simulink model "Pendulum_final"  (R2024b)
settings: Solver=VariableStepAuto  StartTime=0.0  StopTime=10.0  RelTol=1e-3
values from neighbouring files (symbols this model uses):
  K = lqr(A_upper,B_upper,Q,R)    [main_final.m]
  P1 = - 0.7065    (= -0.7065)    [main_final.m]
  P2 = - 1.44    (= -1.44)    [main_final.m]
  P3 = 0.05622    [main_final.m]
  P4 = 0.008979    [main_final.m]
  P5 = 0.00232    [main_final.m]
  P6 = 1    [main_final.m]
  phi_dot_dot_sat = 100    [main_final.m]
  phi_dot_dot_threshold = 1e-10    [main_final.m]
  tau_a_sat = inf    [main_final.m]
  tau_a_threshold = 1e-10    [main_final.m]
  theta_dot_dot_sat = 100    [main_final.m]
  theta_dot_dot_threshold = 1e-10    [main_final.m]
settings Model: Creator=louis  LastModifiedBy=sipak

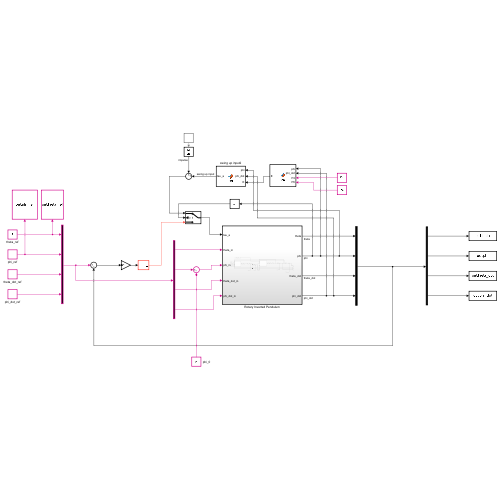
[thumbnail: Simulink's stored preview of the top-level diagram]
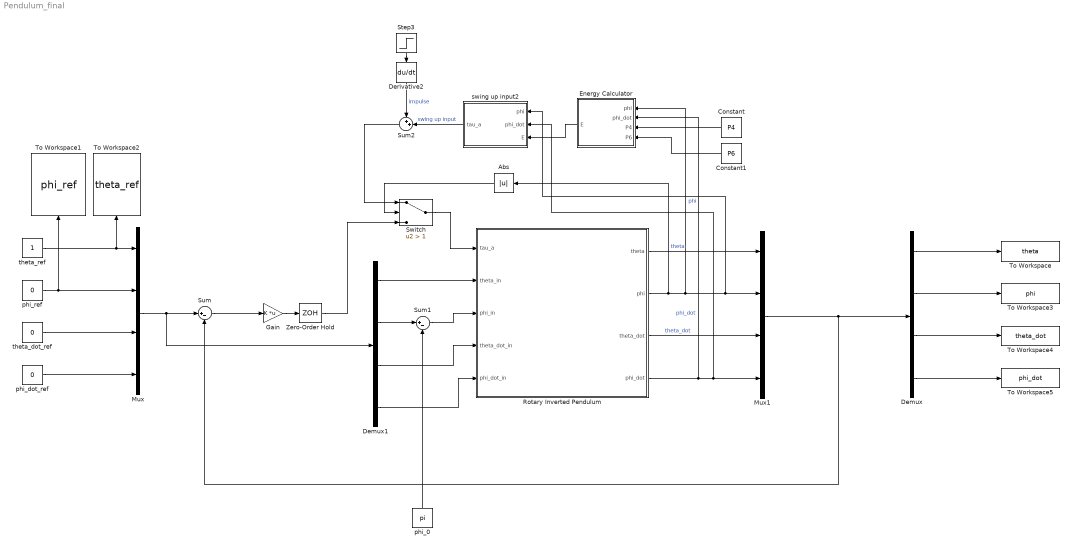
== system Pendulum_final ==
  Abs : Abs  SaturateOnIntegerOverflow=off
  Constant : Constant  Value=P4
  Constant1 : Constant  Value=P6
  Demux : Demux
  Demux1 : Demux
  Derivative2 : Derivative
  Energy Calculator : MATLAB Function  TreatAsAtomicUnit=on
  Gain : Gain  Gain=K  Multiplication=Matrix(K*u)
  Mux : Mux
  Mux1 : Mux
  Rotary Inverted Pendulum : Subsystem
  Step3 : Step  SampleTime=0
  Sum : Sum  Inputs=|+-
  Sum1 : Sum  Inputs=|+-
  Sum2 : Sum  Inputs=++|
  Switch : Switch  Criteria=u2 > Threshold  Threshold=1  SaturateOnIntegerOverflow=off  InputSameDT=off
  To Workspace : ToWorkspace  VariableName=theta  SampleTime=-1
      settings: Save2DSignal=2-D array (concatenate along first dimension)
  To Workspace1 : ToWorkspace  VariableName=phi_ref  SampleTime=-1
      settings: Save2DSignal=2-D array (concatenate along first dimension)
  To Workspace2 : ToWorkspace  VariableName=theta_ref  SampleTime=-1
  To Workspace3 : ToWorkspace  VariableName=phi  SampleTime=-1
  To Workspace4 : ToWorkspace  VariableName=theta_dot  SampleTime=-1
  To Workspace5 : ToWorkspace  VariableName=phi_dot  SampleTime=-1
  Zero-Order Hold : ZeroOrderHold  SampleTime=0.01
  phi_0 : Constant  Value=pi
  phi_dot_ref : Constant  Value=0
  phi_ref : Constant  Value=0
  swing up input2 : MATLAB Function  TreatAsAtomicUnit=on
  theta_dot_ref : Constant  Value=0
  theta_ref : Constant
  wires:
  theta_dot_ref/1 -> Mux/3
  phi_ref/1 -> Mux/2, To Workspace1/1
  theta_ref/1 -> Mux/1, To Workspace2/1
  Gain/1 -> Zero-Order Hold/1
  Mux/1 -> Demux1/1, Sum/1
  Mux1/1 -> Demux/1, Sum/2
  Sum/1 -> Gain/1
  Demux/1 -> To Workspace/1
  Demux/2 -> To Workspace3/1
  Demux/3 -> To Workspace4/1
  Demux/4 -> To Workspace5/1
  Demux1/3 -> Rotary Inverted Pendulum/4(theta_dot_in)
  Demux1/4 -> Rotary Inverted Pendulum/5(phi_dot_in)
  Demux1/1 -> Rotary Inverted Pendulum/2(theta_in)
  Rotary Inverted Pendulum/1(theta) -> Mux1/1  "theta"
  Rotary Inverted Pendulum/2(phi) -> Abs/1, swing up input2/1(phi), Mux1/2, Energy Calculator/1(phi)  "phi"
  Rotary Inverted Pendulum/3(theta_dot) -> Mux1/3  "theta_dot"
  Rotary Inverted Pendulum/4(phi_dot) -> Energy Calculator/2(phi_dot), swing up input2/2(phi_dot), Mux1/4  "phi_dot"
  phi_dot_ref/1 -> Mux/4
  Demux1/2 -> Sum1/1
  Sum1/1 -> Rotary Inverted Pendulum/3(phi_in)
  phi_0/1 -> Sum1/2
  Constant/1 -> Energy Calculator/3(P4)
  Step3/1 -> Derivative2/1
  Constant1/1 -> Energy Calculator/4(P6)
  Energy Calculator/1(E) -> swing up input2/3(E)
  Zero-Order Hold/1 -> Switch/3
  swing up input2/1(tau_a) -> Sum2/2  "swing up input"
  Sum2/1 -> Switch/1
  Switch/1 -> Rotary Inverted Pendulum/1(tau_a)
  Abs/1 -> Switch/2
  Derivative2/1 -> Sum2/1  "impulse"

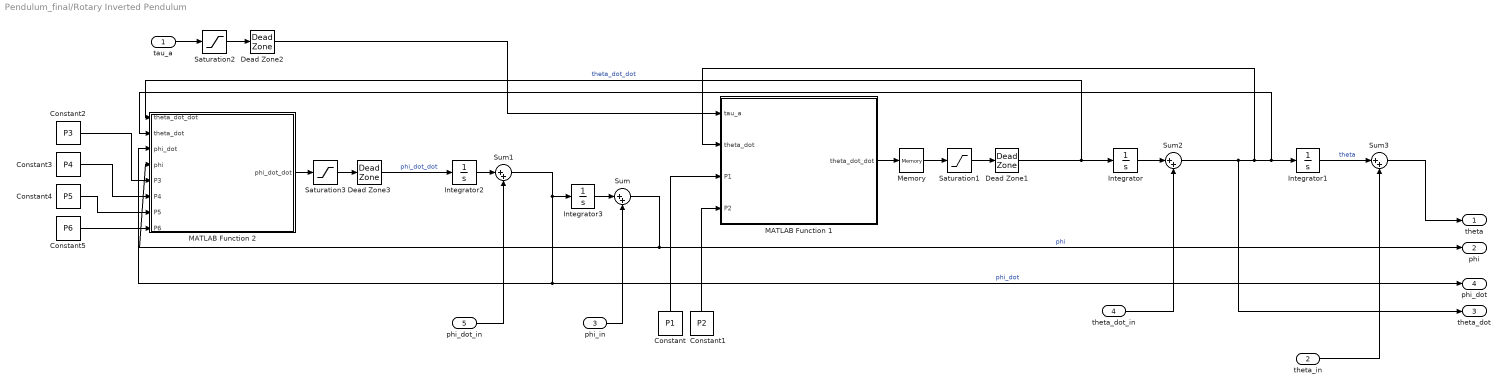
== system Pendulum_final/Rotary Inverted Pendulum ==
  tau_a : Inport
  theta_in : Inport  Port=2
  phi_in : Inport  Port=3
  theta_dot_in : Inport  Port=4
  phi_dot_in : Inport  Port=5
  Constant : Constant  Value=P1
  Constant1 : Constant  Value=P2
  Constant2 : Constant  Value=P3
  Constant3 : Constant  Value=P4
  Constant4 : Constant  Value=P5
  Constant5 : Constant  Value=P6
  Dead Zone1 : DeadZone  LowerValue=-theta_dot_dot_threshold  UpperValue=theta_dot_dot_threshold
  Dead Zone2 : DeadZone  LowerValue=-tau_a_threshold  UpperValue=tau_a_threshold
  Dead Zone3 : DeadZone  LowerValue=-phi_dot_dot_threshold  UpperValue=phi_dot_dot_threshold
  Integrator{,1..3} (4 alike) : Integrator
  MATLAB Function 1 : MATLAB Function  TreatAsAtomicUnit=on
  MATLAB Function 2 : MATLAB Function  TreatAsAtomicUnit=on
  Memory : Memory
  Saturation1 : Saturate  UpperLimit=theta_dot_dot_sat  LowerLimit=-theta_dot_dot_sat
  Saturation2 : Saturate  UpperLimit=tau_a_sat  LowerLimit=-tau_a_sat
  Saturation3 : Saturate  UpperLimit=phi_dot_dot_sat  LowerLimit=-phi_dot_dot_sat
  Sum{,1..3} (4 alike) : Sum  Inputs=|++
  theta : Outport
  phi : Outport  Port=2
  theta_dot : Outport  Port=3
  phi_dot : Outport  Port=4
  wires:
  Integrator2/1 -> Sum1/1
  Integrator/1 -> Sum2/1
  Sum/1 -> phi/1, MATLAB Function 2/4(phi)  "phi"
  MATLAB Function 2/1(phi_dot_dot) -> Saturation3/1
  phi_in/1 -> Sum/2
  tau_a/1 -> Saturation2/1
  Integrator3/1 -> Sum/1
  theta_dot_in/1 -> Sum2/2
  phi_dot_in/1 -> Sum1/2
  MATLAB Function 1/1(theta_dot_dot) -> Memory/1
  Memory/1 -> Saturation1/1
  Sum1/1 -> phi_dot/1, MATLAB Function 2/3(phi_dot), Integrator3/1  "phi_dot"
  Sum2/1 -> MATLAB Function 1/2(theta_dot), MATLAB Function 2/2(theta_dot), Integrator1/1, theta_dot/1
  Saturation2/1 -> Dead Zone2/1
  Dead Zone2/1 -> MATLAB Function 1/1(tau_a)
  Dead Zone3/1 -> Integrator2/1  "phi_dot_dot"
  Saturation3/1 -> Dead Zone3/1
  Saturation1/1 -> Dead Zone1/1
  Dead Zone1/1 -> MATLAB Function 2/1(theta_dot_dot), Integrator/1  "theta_dot_dot"
  Constant2/1 -> MATLAB Function 2/5(P3)
  Constant4/1 -> MATLAB Function 2/7(P5)
  Constant3/1 -> MATLAB Function 2/6(P4)
  Constant5/1 -> MATLAB Function 2/8(P6)
  Constant/1 -> MATLAB Function 1/3(P1)
  Constant1/1 -> MATLAB Function 1/4(P2)
  theta_in/1 -> Sum3/2
  Integrator1/1 -> Sum3/1  "theta"
  Sum3/1 -> theta/1

== matlab function Pendulum_final/Rotary Inverted Pendulum/MATLAB Function 2 ==
  data: theta_dot_dot input; phi_dot_dot output; theta_dot input; phi_dot input; phi input; P3 input; P4 input; P5 input; P6 input
function phi_dot_dot = equation2(theta_dot_dot, theta_dot, phi_dot, phi, P3, P4, P5, P6)

    tau_p = 0;
    phi_dot_dot = (2 * tau_p - (P3 * theta_dot_dot * cos(phi)) ...
                   + (0 * theta_dot^2 * sin(2 * phi)) ... % We put 0 times the rest because Ip_y2 disappear when linearizing. That might be false
                   + (P6 * sin(phi)) ...
                   - (P5 * phi_dot)) / P4;
end

== matlab function Pendulum_final/Rotary Inverted Pendulum/MATLAB Function 1 ==
  data: tau_a input; theta_dot_dot output; theta_dot input; P1 input; P2 input
function theta_dot_dot = equation1(tau_a, theta_dot, P1, P2)

    theta_dot_dot = (tau_a - (P2 * theta_dot)) / P1;
    
end

== matlab function Pendulum_final/Energy Calculator ==
  data: phi input; phi_dot input; P4 input; E output; P6 input
function E = fcn(phi, phi_dot, P4, P6)
    % P4 = 2 * Ip_x2
    % P6 = mp * g * l

    omega0 = sqrt(P6 / (P4/2));
    E = P6 * (0.5 * (phi_dot / omega0)^2 + cos(phi) - 1);
    
end

== matlab function Pendulum_final/swing up input2 ==
  data: phi input; phi_dot input; E input; tau_a output
function tau_a = fcn(phi, phi_dot, E)
    k_swing = 2;
    E_target = 0;
    tau_a = k_swing * (E_target-E) * sign(phi_dot * cos(phi));
end
